simulink model "SystemLoopDiscrete"  (R2023a)
settings: Solver=FixedStepAuto  StartTime=0.0  StopTime=20  RelTol=1e-3  EnableMultiTasking=on
values from neighbouring files (symbols this model uses):
  L = 8.2*10^(-3)    (= 0.0082)    [phaseplane.m]
undefined symbols (not defined in the file or in its folder): Ad, Bd, Cd, Dd, DiscIntNeverNeededParam, ki, Kp, Ts
libraries: mbedblockslib x3, stm_qeplib x1
settings Model: ExtModeTrigDuration=10  Creator=Marco  LastModifiedBy=Marco
settings OptimizationCC: EnhancedBackFolding=on  PassReuseOutputArgsAs=Individual arguments  ZeroExternalMemoryAtStartup=off  ZeroInternalMemoryAtStartup=off  MaxStackSize=64  OptimizeBlockOrder=speed  DifferentSizesBufferReuse=on  OptimizationCustomize=off  EfficientTunableParamExpr=on
settings DebuggingCC: ParameterTunabilityLossMsg=error
settings HardwareCC: ProdBitPerPointer=32  ProdBitPerSizeT=32  ProdBitPerPtrDiffT=32  ProdLargestAtomicInteger=Long  ProdLargestAtomicFloat=Double  ProdWordSize=32  ProdLongLongMode=on  ProdHWDeviceType=ARM Compatible->ARM Cortex
settings SFSimCC: MATLABDynamicMemAlloc=off
settings RTWCC: Description=Embedded Coder  SystemTargetFile=ert.tlc  HardwareBoard=STM32 Nucleo F401RE  TemplateMakefile=ert_default_tmf  Toolchain=GNU Tools for ARM Embedded Processors
settings CodeAppCC: ForceParamTrailComments=on  IgnoreCustomStorageClasses=off  OperatorAnnotations=on  SimulinkDataObjDesc=on  SFDataObjDesc=on  InsertBlockDesc=on
settings ERTTargetCC: ExtModeTransport=3  ExtModeStaticAlloc=on  ExtModeStaticAllocSize=2000  ExtModeMexFile=ext_xcp  ExtModeIntrfLevel=Level2 - Open

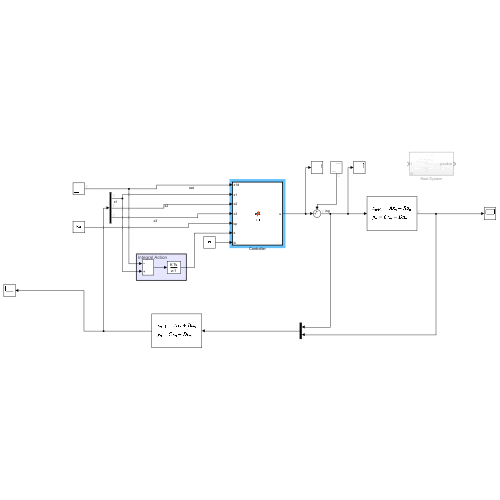
[thumbnail: Simulink's stored preview of the top-level diagram]
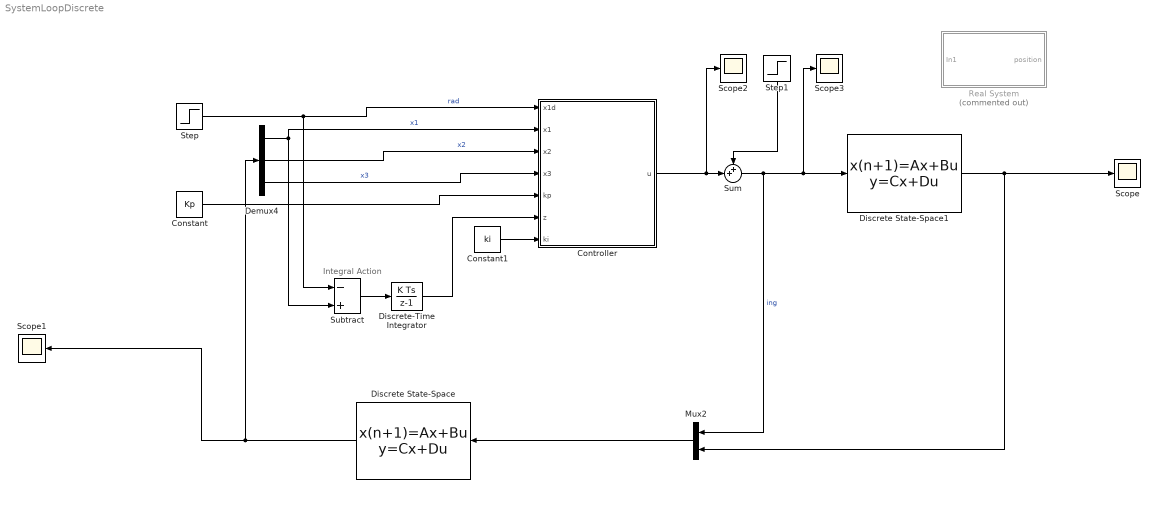
== system SystemLoopDiscrete ==
  note: Integral Action
  Constant : Constant  Value=Kp  SampleTime=Ts
  Constant1 : Constant  Value=ki  SampleTime=Ts
  Controller : MATLAB Function  TreatAsAtomicUnit=on
  Demux4 : Demux  Outputs=3
  Discrete State-Space : DiscreteStateSpace  A=Ad-L*Cd  B=[Bd L]  C=eye(3)  D=[ 0 0; 0 0; 0 0]  SampleTime=Ts
  Discrete State-Space1 : DiscreteStateSpace  A=Ad  B=Bd  C=Cd  D=Dd  SampleTime=Ts
  Discrete-Time Integrator : DiscreteIntegrator  gainval=1  SampleTime=Ts  ICPrevOutput=DiscIntNeverNeededParam  ICPrevScaledInput=DiscIntNeverNeededParam
  Mux2 : Mux  Inputs=2
  Real System : Subsystem  Commented=on
  Scope{,1..3} (4 alike) : Scope
  Step : Step  Time=0  SampleTime=Ts
  Step1 : Step  Time=0  After=0  SampleTime=Ts
  Subtract : Sum  Inputs=-+
  Sum : Sum  Inputs=++|
  wires:
  Discrete State-Space/1 -> Demux4/1, Scope1/1
  Mux2/1 -> Discrete State-Space/1
  Demux4/2 -> Controller/3(x2)  "x2"
  Demux4/3 -> Controller/4(x3)  "x3"
  Step1/1 -> Sum/1
  Sum/1 -> Discrete State-Space1/1, Scope3/1, Mux2/1  "ing"
  Discrete-Time Integrator/1 -> Controller/6(z)
  Discrete State-Space1/1 -> Mux2/2, Scope/1
  Constant/1 -> Controller/5(kp)
  Step/1 -> Controller/1(x1d), Subtract/1  "rad"
  Subtract/1 -> Discrete-Time Integrator/1
  Controller/1(u) -> Scope2/1, Sum/2
  Demux4/1 -> Subtract/2, Controller/2(x1)  "x1"
  Constant1/1 -> Controller/7(ki)

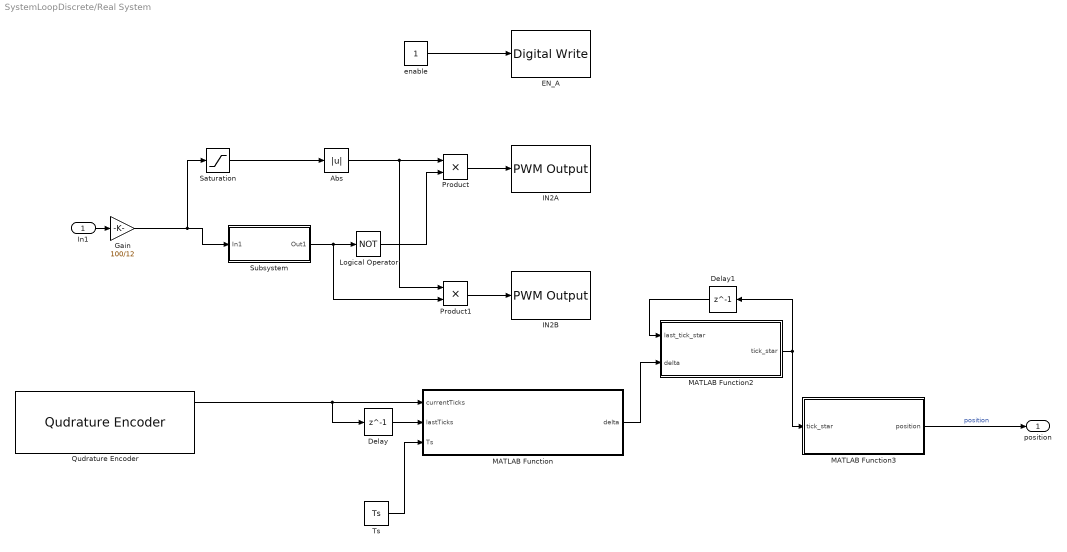
== system SystemLoopDiscrete/Real System ==
  In1 : Inport
  Abs : Abs  SaturateOnIntegerOverflow=off
  Delay : Delay  DelayLength=1  InitialCondition=0
  Delay1 : Delay  DelayLength=1  InitialCondition=0
  EN_A : mbedblockslib/Digital Write  Pin=2  Direction=output
      settings: LibrarySourceBlock=stmnucleorootlib/Common/Digital Write
  Gain : Gain  Gain=100/12
  IN2A : mbedblockslib/PWM Output  Pin=4  EnableInputFrequency=off  InitialFrequency=PWMFreq  InitialDutyCycle=50  NotificationType=None
      settings: LibrarySourceBlock=stmnucleorootlib/Common/PWM Output
  IN2B : mbedblockslib/PWM Output  Pin=5  EnableInputFrequency=off  InitialFrequency=PWMFreq  InitialDutyCycle=50  NotificationType=None
      settings: LibrarySourceBlock=stmnucleorootlib/Common/PWM Output
  Logical Operator : Logic  Operator=NOT  AllPortsSameDT=off  OutDataTypeStr=boolean
  MATLAB Function : MATLAB Function  TreatAsAtomicUnit=on
  MATLAB Function2 : MATLAB Function  TreatAsAtomicUnit=on
  MATLAB Function3 : MATLAB Function  TreatAsAtomicUnit=on
  Product : Product
  Product1 : Product
  Qudrature Encoder : stm_qeplib/Qudrature Encoder  SampleTime=Ts
  Saturation : Saturate  UpperLimit=100  LowerLimit=-100
  Subsystem : Subsystem
  Ts : Constant  Value=Ts
  enable : Constant
  position : Outport
  wires:
  enable/1 -> EN_A/1
  Subsystem/1(Out1) -> Product1/2, Logical Operator/1
  Saturation/1 -> Abs/1
  Product1/1 -> IN2B/1
  Product/1 -> IN2A/1
  Logical Operator/1 -> Product/2
  Abs/1 -> Product1/1, Product/1
  Gain/1 -> Saturation/1, Subsystem/1(In1)
  MATLAB Function2/1(tick_star) -> MATLAB Function3/1(tick_star), Delay1/1
  Qudrature Encoder/1 -> Delay/1, MATLAB Function/1(currentTicks)
  MATLAB Function/1(delta) -> MATLAB Function2/2(delta)
  Delay1/1 -> MATLAB Function2/1(last_tick_star)
  Ts/1 -> MATLAB Function/3(Ts)
  Delay/1 -> MATLAB Function/2(lastTicks)
  In1/1 -> Gain/1
  MATLAB Function3/1(position) -> position/1  "position"

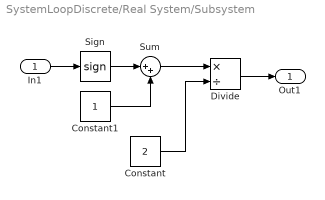
== system SystemLoopDiscrete/Real System/Subsystem ==
  In1 : Inport
  Constant : Constant  Value=2
  Constant1 : Constant
  Divide : Product  Inputs=*/
  Sign : Signum
  Sum : Sum  Inputs=|++
  Out1 : Outport
  wires:
  In1/1 -> Sign/1
  Sign/1 -> Sum/1
  Constant1/1 -> Sum/2
  Sum/1 -> Divide/1
  Constant/1 -> Divide/2
  Divide/1 -> Out1/1

== matlab function SystemLoopDiscrete/Real System/MATLAB Function ==
  data: currentTicks input; delta output; lastTicks input; Ts input
function delta = getTicksDelta(currentTicks, lastTicks, Ts)

currentTicks = double(currentTicks);
lastTicks = double(lastTicks);

if abs(currentTicks - lastTicks) <= ceil(8400*Ts)
    delta = currentTicks-lastTicks;
else
    if lastTicks > currentTicks
        delta = currentTicks + 2^16-1-lastTicks;
    else
        delta = currentTicks - 2^16+1-lastTicks;

end

end

== matlab function SystemLoopDiscrete/Controller ==
  data: x1d input; x1 input; u output; x2 input; x3 input; kp input; z input; ki input
function u = fcn(x1d, x1, x2, x3, kp, z, ki)

c = -kp(1)*(x1-x1d) - kp(2)*x2 - kp(3)*x3 - ki*z;

u = c

== matlab function SystemLoopDiscrete/Real System/MATLAB Function2 ==
  data: last_tick_star input; delta input; tick_star output
function tick_star = modCounter(last_tick_star, delta)

    % 89796 numero di tick per effettuare 25 giri completo
    tick_star = mod(last_tick_star + delta, 89796)

end

== matlab function SystemLoopDiscrete/Real System/MATLAB Function3 ==
  data: tick_star input; position output
function position = getPosition(tick_star)

    tick_star = double(tick_star);

    completeTheta = 2*pi*tick_star/(3591.84);

    position = sign(completeTheta) * mod(abs(completeTheta), 2*pi);

end
